simulink model "MRAC_OF_Non_Linear_Simulink"  (R2018a)
settings: Solver=ode45  StartTime=0.0  StopTime=20*T_Uc  RelTol=1e-3  EnableMultiTasking=on
undefined symbols (not defined in the file): a0, a1, a2, A_ch1, A_ch2, A_p, alfa, Am, am1, am2, Amp_Uc, b, b0, b0_init, bm, C, d, Gamma, gamma1, gamma2, h0_1, h0_2, h1_init, h2_init, l, mu, P, P1, P2, P2_init, P_atm, Ps, R, r1p, r1p_init, Roh_air, Roh_w, s0, s0_init, s1, s1_init, T0, t0, t0_init, T1, t1, t1_init, T2, T_Uc, Tf, Ts
settings Model: Creator=ahmad  LastModifiedBy=Ahmad
settings DataIOCC: LimitDataPoints=on  SaveFormat=Array
settings OptimizationCC: LifeSpan=inf
settings DebuggingCC: UnderspecifiedInitializationDetection=Classic  MergeDetectMultiDrivingBlocksExec=none  SolverPrmCheckMsg=warning  StateNameClashWarn=warning  SFUnexpectedBacktrackingDiag=warning  SFNoUnconditionalDefaultTransitionDiag=warning  SFExecutionAtInitializationDiag=none
settings HardwareCC: ProdBitPerPointer=32  ProdBitPerSizeT=32  ProdBitPerPtrDiffT=32  ProdLargestAtomicFloat=None  ProdIntDivRoundTo=Undefined  ProdEndianess=Unspecified  ProdWordSize=32  ProdHWDeviceType=32-bit Generic
settings ModelReferenceCC: PropagateSignalLabelsOutOfModel=off
settings CodeAppCC: StateflowObjectComments=on
settings GRTTargetCC: TargetLangStandard=C89/C90 (ANSI)  GeneratePreprocessorConditionals=Disable all
settings ConfigComp: CovMetricSettings=dw  CovHtmlReporting=on  CovSaveCumulativeToWorkspaceVar=on  CovSaveSingleToWorkspaceVar=on  CovExternalEMLEnable=off

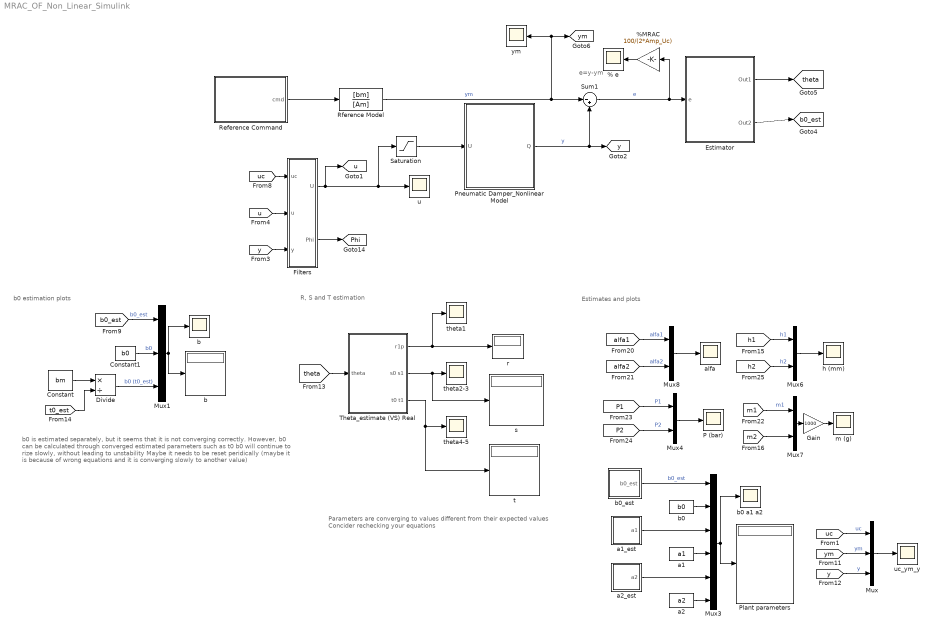
== system MRAC_OF_Non_Linear_Simulink ==
  note: Estimates and plots
  note: R, S and T estimation
  note: b0 estimation plots
  note: Parameters are converging to values different from their expected values
      | Concider rechecking your equations
  note: b0 is estimated separately, but it seems that it is not converging correctly.
      | However, b0 can be calculated through converged estimated parameters such as t0
      |
      | b0 will continue to rize slowly, without leading to unstability
      | Maybe it needs to be reset peridically
      | (maybe it is because of wrong equations and it is converging slowly to another value)
  note: e=y-ym
  % e : Scope
  %MRAC : Gain  Gain=100/(2*Amp_Uc)
  Constant : Constant  Value=bm
  Constant1 : Constant  Value=b0
  Divide : Product  Inputs=*/
  Estimator : Subsystem
  Filters : Subsystem
  Gain : Gain  Gain=1000
  Mux : Mux  Inputs=3
  Mux1 : Mux  Inputs=3
  Mux3 : Mux  Inputs=6
  Mux{4,6..8} (4 alike) : Mux  Inputs=2
  P (bar) : Scope
  Plant parameters : Display
  Pneumatic Damper_Nonlinear Model : Subsystem
  Reference Command : Subsystem
  Rference Model : TransferFcn  Numerator=[bm]  Denominator=[Am]
  Saturation : Saturate  UpperLimit=1  LowerLimit=-1
  Sum1 : Sum  Inputs=|-+
  Theta_estimate (VS) Real : Subsystem
  a1 : Constant  Value=a1
  a1_est : Subsystem
  a2 : Constant  Value=a2
  a2_est : Subsystem
  alfa : Scope
  b : Scope
  "b " : Display
  b0 : Constant  Value=b0
  b0 a1 a2 : Scope
  b0_est : Subsystem
  h (mm) : Scope
  m (g) : Scope
  r : Display
  s : Display
  t : Display
  theta1 : Scope
  theta2-3 : Scope
  theta4-5 : Scope
  u : Scope
  uc_ym_y : Scope
  ym : Scope
  tag scope: Phi=global, b0_est=global, theta=global, u=global, y=global, ym=global
  wires:
  Pneumatic Damper_Nonlinear Model/1("Q  ") -> [y], Sum1/2  "y"
  Rference Model/1 -> Sum1/1, [ym], ym/1  "ym"
  Sum1/1 -> %MRAC/1, Estimator/1(e)  "e"
  Mux/1 -> uc_ym_y/1
  [uc] -> Mux/1  "uc"
  [u] -> Filters/2(u)
  [y] -> Filters/3(y)
  Filters/2(Phi) -> [Phi]
  Mux1/1 -> "b "/1, b/1
  Constant1/1 -> Mux1/2  "b0"
  [b0_est] -> Mux1/1  "b0_est"
  [uc] -> Filters/1(uc)
  Filters/1(U) -> Saturation/1, u/1, [u]
  [y] -> Mux/3  "y"
  [ym] -> Mux/2  "ym"
  Theta_estimate (VS) Real/3(t0	t1) -> t/1, theta4-5/1
  Theta_estimate (VS) Real/2(s0	s1) -> s/1, theta2-3/1
  Theta_estimate (VS) Real/1(r1p) -> theta1/1, r/1
  [theta] -> Theta_estimate (VS) Real/1(theta)
  [t0_est] -> Divide/2
  Constant/1 -> Divide/1
  Divide/1 -> Mux1/3  "b0 (t0_est)"
  Mux3/1 -> b0 a1 a2/1, Plant parameters/1
  b0/1 -> Mux3/2
  a1/1 -> Mux3/4
  b0_est/1(b0_est) -> Mux3/1  "b0_est"
  a1_est/1(a1) -> Mux3/3
  a2_est/1(a2) -> Mux3/5
  a2/1 -> Mux3/6
  %MRAC/1 -> % e/1
  [P1] -> Mux4/1  "P1"
  [P2] -> Mux4/2  "P2"
  Mux4/1 -> P (bar)/1
  [h1] -> Mux6/1  "h1"
  [h2] -> Mux6/2  "h2"
  Mux6/1 -> h (mm)/1
  [m1] -> Mux7/1  "m1"
  [m2] -> Mux7/2
  Mux7/1 -> Gain/1
  Gain/1 -> m (g)/1
  [alfa1] -> Mux8/1  "alfa1"
  [alfa2] -> Mux8/2  "alfa2"
  Mux8/1 -> alfa/1
  Saturation/1 -> Pneumatic Damper_Nonlinear Model/1(U)
  Reference Command/1(cmd) -> Rference Model/1
  Estimator/1(Out1) -> [theta]
  Estimator/2(Out2) -> [b0_est]

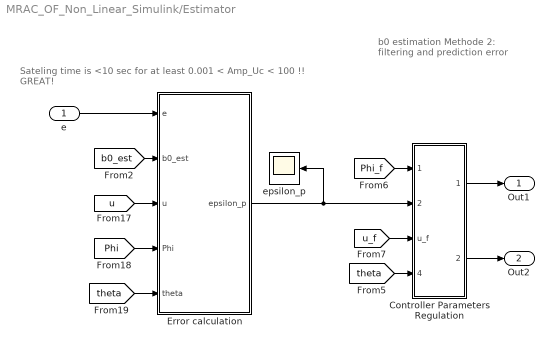
== system MRAC_OF_Non_Linear_Simulink/Estimator ==
  note: b0 estimation
      | Methode 2:
      | filtering and prediction error
  note: Sateling time is <10 sec for at least 0.001 < Amp_Uc < 100 !!
      | GREAT!
  e : Inport
  Controller Parameters Regulation : Subsystem
  Error calculation : Subsystem
  epsilon_p : Scope
  Out1 : Outport
  Out2 : Outport  Port=2
  wires:
  [Phi] -> Error calculation/4("Phi ")
  [b0_est] -> Error calculation/2(b0_est)
  e/1 -> Error calculation/1("e ")
  [u] -> Error calculation/3(u)
  [Phi_f] -> Controller Parameters Regulation/1(Phi_f)
  [u_f] -> Controller Parameters Regulation/3(u_f)
  [theta] -> Error calculation/5(theta)
  Error calculation/1(epsilon_p) -> epsilon_p/1, Controller Parameters Regulation/2(epsilon_p)
  [theta] -> Controller Parameters Regulation/4("theta ")
  Controller Parameters Regulation/2(b0_est) -> Out2/1
  Controller Parameters Regulation/1(theta) -> Out1/1

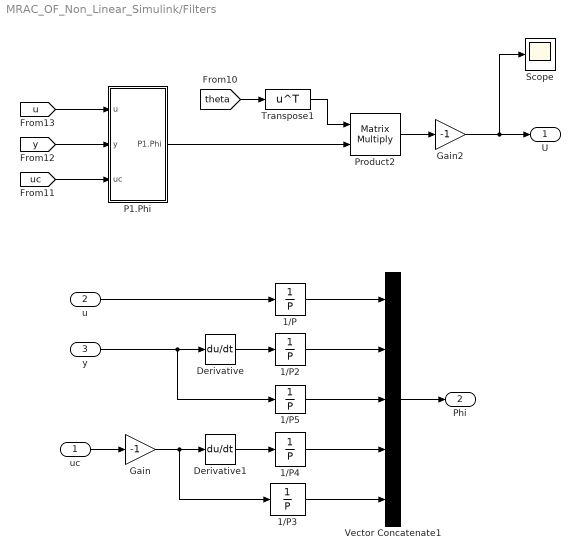
== system MRAC_OF_Non_Linear_Simulink/Filters ==
  uc : Inport
  u : Inport  Port=2
  y : Inport  Port=3
  1/P{,2..5} (5 alike) : TransferFcn  Numerator=1  Denominator=P
  Derivative : Derivative
  Derivative1 : Derivative
  Gain : Gain  Gain=-1
  Gain2 : Gain  Gain=-1
  P1.Phi : Subsystem
  Product2 : Product  Multiplication=Matrix(*)
  Scope : Scope
  Transpose1 : Math  Operator=transpose  SaturateOnIntegerOverflow=on
  Vector Concatenate1 : Concatenate  NumInputs=5
  U : Outport
  Phi : Outport  Port=2
  wires:
  y/1 -> 1/P5/1, Derivative/1
  Derivative1/1 -> 1/P4/1
  1/P3/1 -> Vector Concatenate1/5
  Gain/1 -> 1/P3/1, Derivative1/1
  1/P2/1 -> Vector Concatenate1/2
  Derivative/1 -> 1/P2/1
  1/P4/1 -> Vector Concatenate1/4
  u/1 -> 1/P/1
  Vector Concatenate1/1 -> Phi/1
  1/P5/1 -> Vector Concatenate1/3
  uc/1 -> Gain/1
  1/P/1 -> Vector Concatenate1/1
  [u] -> P1.Phi/1(u)
  [y] -> P1.Phi/2(y)
  [uc] -> P1.Phi/3(uc)
  P1.Phi/1(P1.Phi) -> Product2/2
  Transpose1/1 -> Product2/1
  [theta] -> Transpose1/1
  Product2/1 -> Gain2/1
  Gain2/1 -> Scope/1, U/1

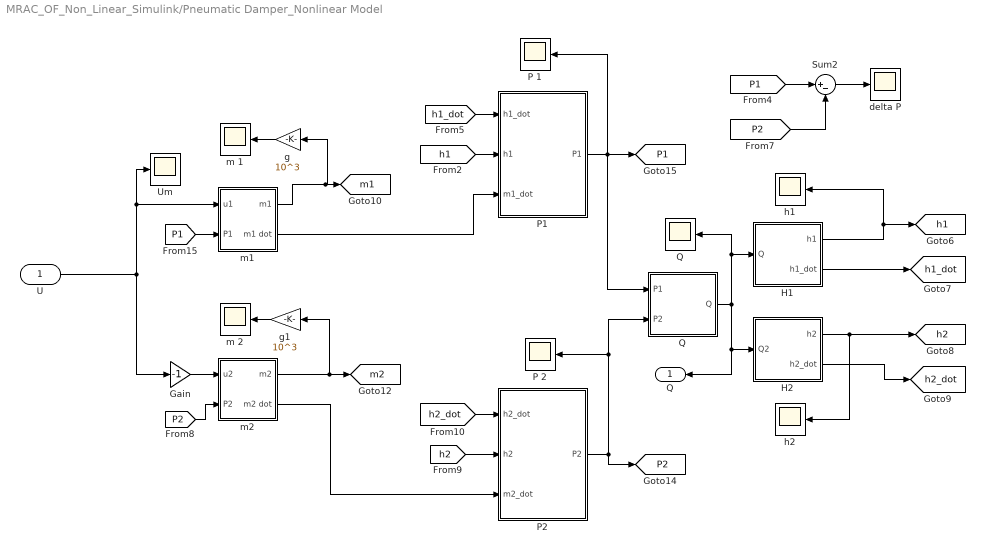
== system MRAC_OF_Non_Linear_Simulink/Pneumatic Damper_Nonlinear Model ==
  U : Inport
  Gain : Gain  Gain=-1
  H1 : Subsystem
  H2 : Subsystem
  P 1 : Scope
  P 2 : Scope
  P1 : Subsystem
  P2 : Subsystem
  Q : Subsystem
  "Q " : Scope
  Sum2 : Sum  Inputs=|+-
  Um : Scope
  delta P : Scope
  g : Gain  Gain=10^3
  g1 : Gain  Gain=10^3
  h1 : Scope
  h2 : Scope
  m 1 : Scope
  m 2 : Scope
  m1 : Subsystem
  m2 : Subsystem
  "Q  " : Outport
  tag scope: P1=global, P2=global, h1=global, h1_dot=global, h2=global, h2_dot=global, m1=global, m2=global
  wires:
  H1/1(h1) -> [h1], h1/1
  H1/2(h1_dot) -> [h1_dot]
  H2/2(h2_dot) -> [h2_dot]
  H2/1(h2) -> h2/1, [h2]
  m1/1(m1) -> g/1, [m1]
  m2/1(m2) -> g1/1, [m2]
  m2/2(m2 dot) -> P2/3(m2_dot)
  [h2_dot] -> P2/1(h2_dot)
  [h1] -> P1/2(h1)
  [h2] -> P2/2(h2)
  P2/1(P2) -> [P2], P 2/1, Q/2(P2)
  U/1 -> Um/1, m1/1(u1), Gain/1
  P1/1(P1) -> P 1/1, Q/1(P1), [P1]
  Gain/1 -> m2/1(u2)
  Q/1(Q) -> "Q  "/1, H2/1(Q2), H1/1(Q), "Q "/1
  [h1_dot] -> P1/1(h1_dot)
  g/1 -> m 1/1
  [P1] -> Sum2/1
  Sum2/1 -> delta P/1
  [P2] -> Sum2/2
  m1/2(m1 dot) -> P1/3(m1_dot)
  [P2] -> m2/2(P2)
  g1/1 -> m 2/1
  [P1] -> m1/2(P1)

== system MRAC_OF_Non_Linear_Simulink/Reference Command ==
  note: without the Uc filter, the parameters do not converge properly!
  note: Assign  Amp_U from the MATLAB script only!
      | gamma and alfa are based on its value!!
  Constant2 : Constant  Value=gamma1
  Constant3 : Constant  Value=alfa
  Input signal (Uc) : DiscretePulseGenerator  PulseType=Time based  Amplitude=-Amp_Uc  Period=T_Uc  PulseWidth=50  PhaseDelay=T_Uc/2
  "Input signal (Uc) Amp_Uc T_uc " : DiscretePulseGenerator  PulseType=Time based  Amplitude=Amp_Uc  Period=T_Uc  PulseWidth=50
  Mux2 : Mux  Inputs=2
  Sum2 : Sum  Inputs=|++
  Uc filter : TransferFcn  Denominator=conv(conv([T_Uc/100 1],[T_Uc/100 1]),[T_Uc/100 1])
  gamma alfa : Display
  uc : Scope
  cmd : Outport
  tag scope: uc=global
  wires:
  Constant2/1 -> Mux2/1
  Input signal (Uc)/1 -> Sum2/1
  Mux2/1 -> gamma alfa/1
  Uc filter/1 -> cmd/1, [uc], uc/1
  Constant3/1 -> Mux2/2
  Sum2/1 -> Uc filter/1
  "Input signal (Uc) Amp_Uc T_uc "/1 -> Sum2/2

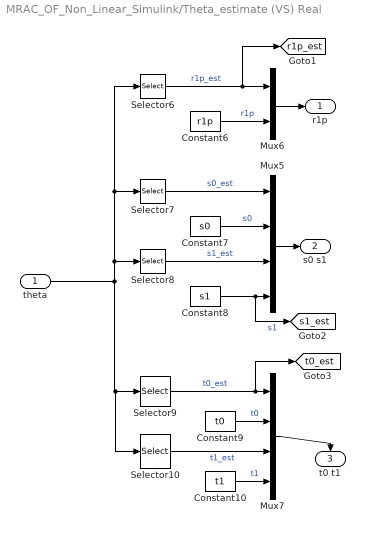
== system MRAC_OF_Non_Linear_Simulink/Theta_estimate (VS) Real ==
  theta : Inport
  Constant10 : Constant  Value=t1
  Constant6 : Constant  Value=r1p
  Constant7 : Constant  Value=s0
  Constant8 : Constant  Value=s1
  Constant9 : Constant  Value=t0
  Mux5 : Mux
  Mux6 : Mux  Inputs=2
  Mux7 : Mux
  Selector10 : Selector  InputPortWidth=5  IndexOptions=Index vector (dialog)  Indices=[5]  OutputSizes=1
  Selector6 : Selector  InputPortWidth=5  IndexOptions=Index vector (dialog)  Indices=[1]  OutputSizes=1
  Selector7 : Selector  InputPortWidth=5  IndexOptions=Index vector (dialog)  Indices=[2]  OutputSizes=1
  Selector8 : Selector  InputPortWidth=5  IndexOptions=Index vector (dialog)  Indices=[3]  OutputSizes=1
  Selector9 : Selector  InputPortWidth=5  IndexOptions=Index vector (dialog)  Indices=[4]  OutputSizes=1
  r1p : Outport
  s0	s1 : Outport  Port=2
  t0	t1 : Outport  Port=3
  tag scope: r1p_est=global, s1_est=global, t0_est=global
  wires:
  Selector7/1 -> Mux5/1  "s0_est"
  Selector6/1 -> [r1p_est], Mux6/1  "r1p_est"
  Mux5/1 -> s0	s1/1
  Selector8/1 -> Mux5/3  "s1_est"
  Constant8/1 -> [s1_est], Mux5/4  "s1"
  Selector9/1 -> [t0_est], Mux7/1  "t0_est"
  Selector10/1 -> Mux7/3  "t1_est"
  Constant10/1 -> Mux7/4  "t1"
  Mux7/1 -> t0	t1/1
  Constant6/1 -> Mux6/2  "r1p"
  theta/1 -> Selector8/1, Selector6/1, Selector7/1, Selector10/1, Selector9/1
  Constant7/1 -> Mux5/2  "s0"
  Constant9/1 -> Mux7/2  "t0"
  Mux6/1 -> r1p/1

== system MRAC_OF_Non_Linear_Simulink/a1_est ==
  Constant4 : Constant  Value=am1
  Sum2 : Sum  Inputs=|-+
  a1 : Outport
  wires:
  Constant4/1 -> Sum2/2
  [r1p_est] -> Sum2/1
  Sum2/1 -> a1/1  "a1"

== system MRAC_OF_Non_Linear_Simulink/a2_est ==
  Constant1 : Constant  Value=am2*a0
  Constant4 : Constant  Value=a0
  Divide1 : Product  Inputs=**
  Divide2 : Product  Inputs=*/
  Sum1 : Sum  Inputs=|+-
  Sum2 : Sum  Inputs=|++
  a2 : Outport
  wires:
  Constant4/1 -> Sum2/2
  [r1p_est] -> Sum2/1
  [s1_est] -> Divide1/1
  [b0_t0_est] -> Divide1/2
  Divide1/1 -> Sum1/2
  Constant1/1 -> Sum1/1
  Sum1/1 -> Divide2/1
  Sum2/1 -> Divide2/2  "r1"
  Divide2/1 -> a2/1  "a2"

== system MRAC_OF_Non_Linear_Simulink/b0_est ==
  Constant4 : Constant  Value=bm
  Divide1 : Product  Inputs=*/
  b0_est : Outport
  tag scope: b0_t0_est=global
  wires:
  [t0_est] -> Divide1/2
  Divide1/1 -> [b0_t0_est], b0_est/1  "b0 (t0_est)"
  Constant4/1 -> Divide1/1

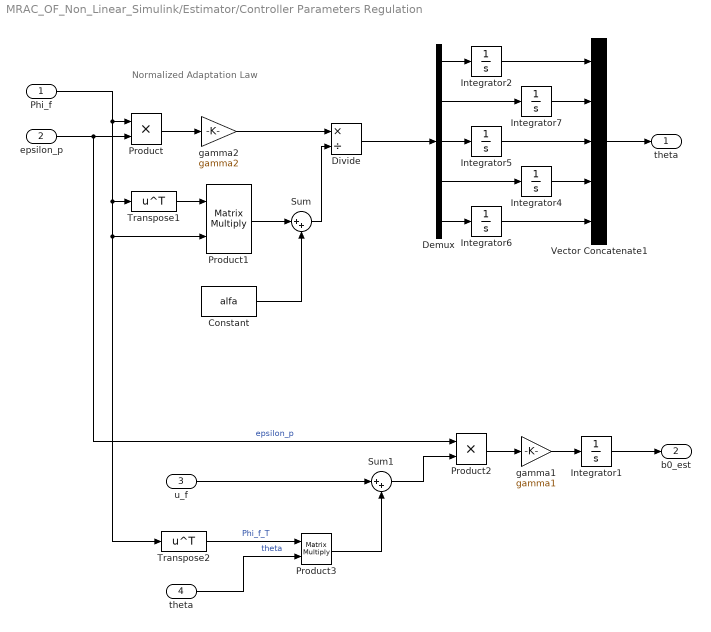
== system MRAC_OF_Non_Linear_Simulink/Estimator/Controller Parameters Regulation ==
  note: Normalized Adaptation Law
  Phi_f : Inport
  epsilon_p : Inport  Port=2
  u_f : Inport  Port=3
  "theta " : Inport  Port=4
  Constant : Constant  Value=alfa
  Demux : Demux  Outputs=5
  Divide : Product  Inputs=*/
  Integrator1 : Integrator  InitialCondition=b0_init
  Integrator2 : Integrator  InitialCondition=r1p_init
  Integrator4 : Integrator  InitialCondition=t0_init
  Integrator5 : Integrator  InitialCondition=s1_init
  Integrator6 : Integrator  InitialCondition=t1_init
  Integrator7 : Integrator  InitialCondition=s0_init
  Product : Product
  Product1 : Product  Multiplication=Matrix(*)
  Product2 : Product
  Product3 : Product  Multiplication=Matrix(*)
  Sum : Sum  Inputs=|++
  Sum1 : Sum  Inputs=|++
  Transpose1 : Math  Operator=transpose  SaturateOnIntegerOverflow=on
  Transpose2 : Math  Operator=transpose  SaturateOnIntegerOverflow=on
  Vector Concatenate1 : Concatenate  NumInputs=5
  gamma1 : Gain  Gain=gamma1
  "gamma2 " : Gain  Gain=gamma2
  theta : Outport
  b0_est : Outport  Port=2
  wires:
  Integrator2/1 -> Vector Concatenate1/1
  Vector Concatenate1/1 -> theta/1
  epsilon_p/1 -> Product2/1, Product/2  "epsilon_p"
  "gamma2 "/1 -> Divide/1
  Demux/4 -> Integrator4/1
  Demux/5 -> Integrator6/1
  Integrator5/1 -> Vector Concatenate1/3
  Integrator4/1 -> Vector Concatenate1/4
  Demux/3 -> Integrator5/1
  Integrator7/1 -> Vector Concatenate1/2
  Integrator6/1 -> Vector Concatenate1/5
  Demux/1 -> Integrator2/1
  Demux/2 -> Integrator7/1
  Phi_f/1 -> Transpose2/1, Product1/2, Transpose1/1, Product/1
  Product/1 -> "gamma2 "/1
  Transpose1/1 -> Product1/1
  Product1/1 -> Sum/1
  Constant/1 -> Sum/2
  Sum/1 -> Divide/2
  Divide/1 -> Demux/1
  u_f/1 -> Sum1/1
  Product2/1 -> gamma1/1
  gamma1/1 -> Integrator1/1
  Integrator1/1 -> b0_est/1
  Transpose2/1 -> Product3/1  "Phi_f_T"
  "theta "/1 -> Product3/2  "theta"
  Product3/1 -> Sum1/2
  Sum1/1 -> Product2/2

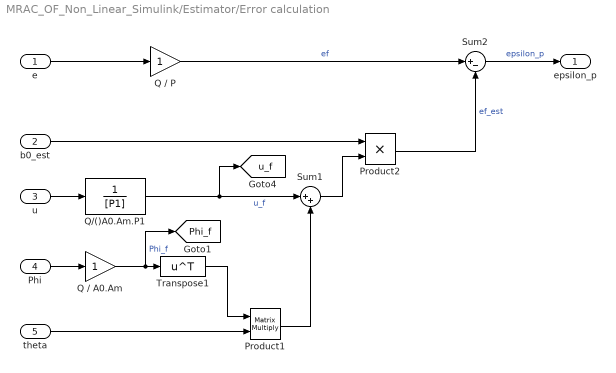
== system MRAC_OF_Non_Linear_Simulink/Estimator/Error calculation ==
  "e " : Inport
  b0_est : Inport  Port=2
  u : Inport  Port=3
  "Phi " : Inport  Port=4
  theta : Inport  Port=5
  Product1 : Product  Multiplication=Matrix(*)
  Product2 : Product
  "Q / A0.Am " : Gain
  Q / P : Gain
  Q/()A0.Am.P1 : TransferFcn  Denominator=[P1]
  Sum1 : Sum  Inputs=|++
  Sum2 : Sum  Inputs=|+-
  Transpose1 : Math  Operator=transpose  SaturateOnIntegerOverflow=on
  epsilon_p : Outport
  tag scope: Phi_f=global, u_f=global
  wires:
  "e "/1 -> Q / P/1
  Q / P/1 -> Sum2/1  "ef"
  Sum2/1 -> epsilon_p/1  "epsilon_p"
  b0_est/1 -> Product2/1
  u/1 -> Q/()A0.Am.P1/1
  Q/()A0.Am.P1/1 -> [u_f], Sum1/1  "u_f"
  "Phi "/1 -> "Q / A0.Am "/1
  "Q / A0.Am "/1 -> [Phi_f], Transpose1/1  "Phi_f"
  Transpose1/1 -> Product1/1
  theta/1 -> Product1/2
  Product1/1 -> Sum1/2
  Sum1/1 -> Product2/2
  Product2/1 -> Sum2/2  "ef_est"

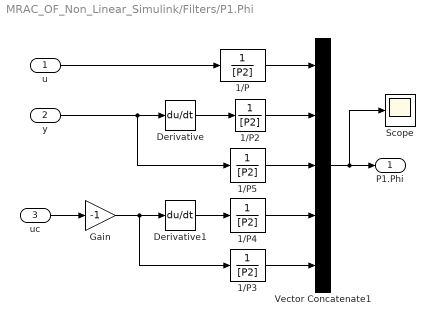
== system MRAC_OF_Non_Linear_Simulink/Filters/P1.Phi ==
  u : Inport
  y : Inport  Port=2
  uc : Inport  Port=3
  1/P{,2..5} (5 alike) : TransferFcn  Numerator=1  Denominator=[P2]
  Derivative : Derivative
  Derivative1 : Derivative
  Gain : Gain  Gain=-1
  Scope : Scope
  Vector Concatenate1 : Concatenate  NumInputs=5
  P1.Phi : Outport
  wires:
  y/1 -> 1/P5/1, Derivative/1
  Derivative1/1 -> 1/P4/1
  1/P3/1 -> Vector Concatenate1/5
  Gain/1 -> 1/P3/1, Derivative1/1
  1/P2/1 -> Vector Concatenate1/2
  Derivative/1 -> 1/P2/1
  1/P4/1 -> Vector Concatenate1/4
  u/1 -> 1/P/1
  1/P5/1 -> Vector Concatenate1/3
  uc/1 -> Gain/1
  1/P/1 -> Vector Concatenate1/1
  Vector Concatenate1/1 -> Scope/1, P1.Phi/1

== system MRAC_OF_Non_Linear_Simulink/Pneumatic Damper_Nonlinear Model/H1 ==
  Q : Inport
  Constant : Constant  Value=A_ch1
  Divide : Product  Inputs=*/
  Integrator : Integrator  InitialCondition=h1_init
  cm-mm : Gain  Gain=-10^3
  h1 : Outport
  h1_dot : Outport  Port=2
  wires:
  Q/1 -> Divide/1
  Integrator/1 -> h1/1  "h1"
  cm-mm/1 -> h1_dot/1, Integrator/1  "h1_dot"
  Divide/1 -> cm-mm/1
  Constant/1 -> Divide/2

== system MRAC_OF_Non_Linear_Simulink/Pneumatic Damper_Nonlinear Model/H2 ==
  Q2 : Inport
  A_pressure_chamber2 : Constant  Value=A_ch2
  Divide : Product  Inputs=*/
  Integrator : Integrator  InitialCondition=h2_init
  cm-mm : Gain  Gain=10^3
  h2 : Outport
  h2_dot : Outport  Port=2
  wires:
  A_pressure_chamber2/1 -> Divide/2
  Q2/1 -> Divide/1
  Integrator/1 -> h2/1  "h2"
  Divide/1 -> cm-mm/1  "h2_dot"
  cm-mm/1 -> Integrator/1, h2_dot/1

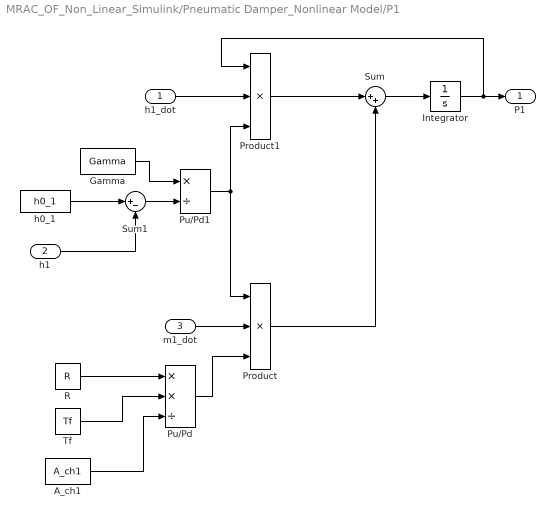
== system MRAC_OF_Non_Linear_Simulink/Pneumatic Damper_Nonlinear Model/P1 ==
  h1_dot : Inport
  h1 : Inport  Port=2
  m1_dot : Inport  Port=3
  A_ch1 : Constant  Value=A_ch1
  Gamma : Constant  Value=Gamma
  Integrator : Integrator  InitialCondition=P2_init
  Product : Product  Inputs=3
  Product1 : Product  Inputs=3
  Pu/Pd : Product  Inputs=**/
  Pu/Pd1 : Product  Inputs=*/
  R : Constant  Value=R
  Sum : Sum  Inputs=|++
  Sum1 : Sum  Inputs=|+-
  Tf : Constant  Value=Tf
  h0_1 : Constant  Value=h0_1
  P1 : Outport
  wires:
  R/1 -> Pu/Pd/1
  A_ch1/1 -> Pu/Pd/3
  Gamma/1 -> Pu/Pd1/1
  Sum1/1 -> Pu/Pd1/2
  h0_1/1 -> Sum1/1
  Tf/1 -> Pu/Pd/2
  Pu/Pd1/1 -> Product/1, Product1/3
  Pu/Pd/1 -> Product/3
  Sum/1 -> Integrator/1
  Integrator/1 -> Product1/1, P1/1
  Product1/1 -> Sum/1
  Product/1 -> Sum/2
  h1_dot/1 -> Product1/2
  h1/1 -> Sum1/2
  m1_dot/1 -> Product/2

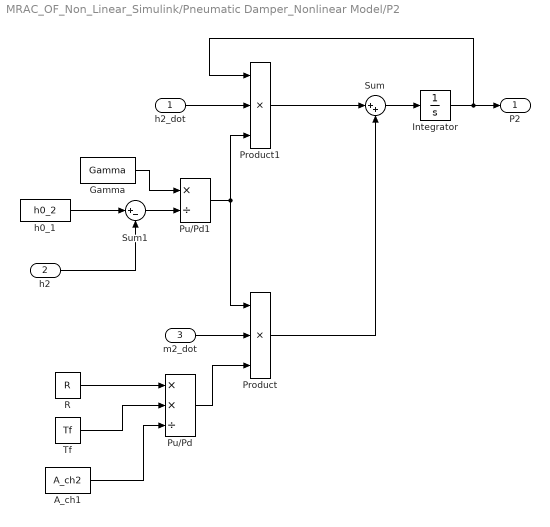
== system MRAC_OF_Non_Linear_Simulink/Pneumatic Damper_Nonlinear Model/P2 ==
  h2_dot : Inport
  h2 : Inport  Port=2
  m2_dot : Inport  Port=3
  A_ch1 : Constant  Value=A_ch2
  Gamma : Constant  Value=Gamma
  Integrator : Integrator  InitialCondition=P2_init
  Product : Product  Inputs=3
  Product1 : Product  Inputs=3
  Pu/Pd : Product  Inputs=**/
  Pu/Pd1 : Product  Inputs=*/
  R : Constant  Value=R
  Sum : Sum  Inputs=|++
  Sum1 : Sum  Inputs=|+-
  Tf : Constant  Value=Tf
  h0_1 : Constant  Value=h0_2
  P2 : Outport
  wires:
  R/1 -> Pu/Pd/1
  A_ch1/1 -> Pu/Pd/3
  Integrator/1 -> Product1/1, P2/1
  Gamma/1 -> Pu/Pd1/1
  Sum1/1 -> Pu/Pd1/2
  h0_1/1 -> Sum1/1
  Tf/1 -> Pu/Pd/2
  Pu/Pd1/1 -> Product/1, Product1/3
  Pu/Pd/1 -> Product/3
  Sum/1 -> Integrator/1
  Product1/1 -> Sum/1
  Product/1 -> Sum/2
  h2_dot/1 -> Product1/2
  h2/1 -> Sum1/2
  m2_dot/1 -> Product/2

== system MRAC_OF_Non_Linear_Simulink/Pneumatic Damper_Nonlinear Model/Q ==
  P1 : Inport
  P2 : Inport  Port=2
  Integrator : Integrator
  Product1 : Product
  Product2 : Product
  Q 2 : Scope
  Sum : Sum  Inputs=|+-
  Sum1 : Sum  Inputs=|+-
  c 4 : Gain  Gain=10^8
  c 5 : Gain  Gain=10^11
  c4 : Subsystem
  c5 : Subsystem
  Q : Outport
  wires:
  P1/1 -> Sum/1
  P2/1 -> Sum/2
  Sum/1 -> Product1/2
  Product1/1 -> Sum1/1
  Integrator/1 -> Q 2/1, Product2/2, Q/1  "Q"
  Product2/1 -> Sum1/2
  Sum1/1 -> Integrator/1
  c4/1(c4) -> c 4/1
  c 4/1 -> Product1/1
  c 5/1 -> Product2/1
  c5/1(c5) -> c 5/1

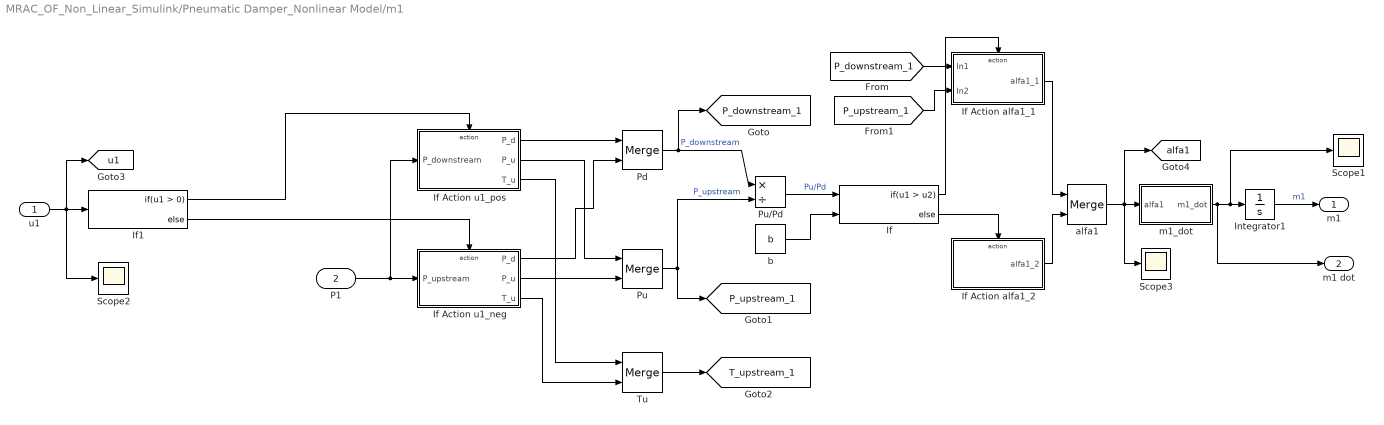
== system MRAC_OF_Non_Linear_Simulink/Pneumatic Damper_Nonlinear Model/m1 ==
  u1 : Inport
  P1 : Inport  Port=2
  If : If  NumInputs=2  IfExpression=u1 > u2
  If Action alfa1_1 : Subsystem  TreatAsAtomicUnit=on
  If Action alfa1_2 : Subsystem  TreatAsAtomicUnit=on
  If Action u1_neg : Subsystem  TreatAsAtomicUnit=on
  If Action u1_pos : Subsystem  TreatAsAtomicUnit=on
  If1 : If
  Integrator1 : Integrator
  Pd : Merge
  Pu : Merge
  Pu/Pd : Product  Inputs=*/
  Scope1 : Scope
  Scope2 : Scope
  Scope3 : Scope
  Tu : Merge
  alfa1 : Merge
  b : Constant  Value=b
  m1_dot : Subsystem
  m1 : Outport
  m1 dot : Outport  Port=2
  tag scope: P_downstream_1=global, P_upstream_1=global, T_upstream_1=global, alfa1=global, u1=global
  wires:
  alfa1/1 -> [alfa1], Scope3/1, m1_dot/1(alfa1)
  Integrator1/1 -> m1/1  "m1"
  If1/2 -> If Action u1_neg/Action
  u1/1 -> Scope2/1, [u1], If1/1
  If1/1 -> If Action u1_pos/Action
  Pu/Pd/1 -> If/1  "Pu/Pd"
  If/1 -> If Action alfa1_1/Action
  If/2 -> If Action alfa1_2/Action
  b/1 -> If/2
  Pd/1 -> Pu/Pd/1, [P_downstream_1]  "P_downstream"
  Pu/1 -> Pu/Pd/2, [P_upstream_1]  "P_upstream"
  If Action u1_pos/1(P_d) -> Pd/1
  If Action alfa1_2/1(alfa1_2) -> alfa1/2
  If Action alfa1_1/1(alfa1_1) -> alfa1/1
  If Action u1_neg/1(P_d) -> Pd/2
  If Action u1_pos/2(P_u) -> Pu/1
  If Action u1_neg/2(P_u) -> Pu/2
  m1_dot/1(m1_dot) -> m1 dot/1, Scope1/1, Integrator1/1
  If Action u1_neg/3(T_u) -> Tu/2
  If Action u1_pos/3(T_u) -> Tu/1
  Tu/1 -> [T_upstream_1]
  [P_downstream_1] -> If Action alfa1_1/1(In1)
  [P_upstream_1] -> If Action alfa1_1/2(In2)
  P1/1 -> If Action u1_pos/1(P_downstream), If Action u1_neg/1(P_upstream)

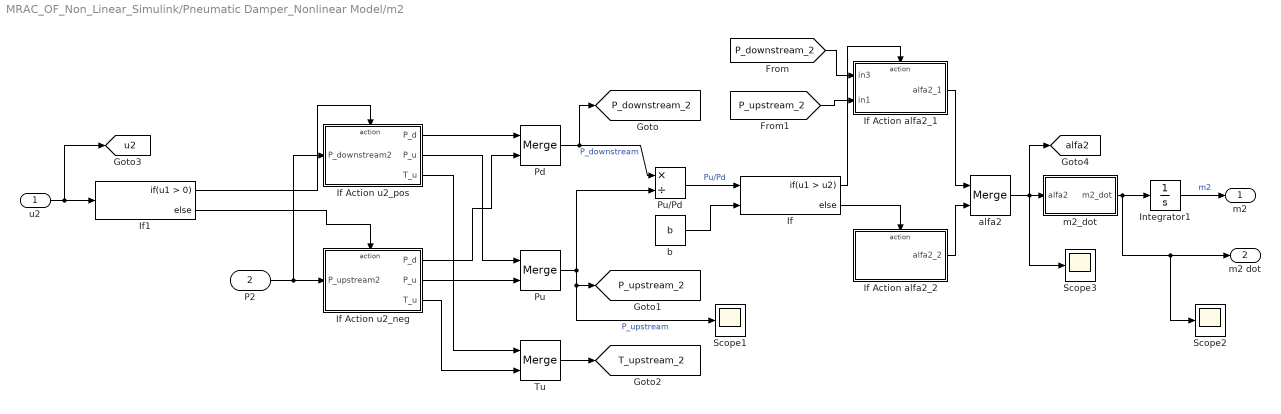
== system MRAC_OF_Non_Linear_Simulink/Pneumatic Damper_Nonlinear Model/m2 ==
  u2 : Inport
  P2 : Inport  Port=2
  If : If  NumInputs=2  IfExpression=u1 > u2
  If Action alfa2_1 : Subsystem  TreatAsAtomicUnit=on
  If Action alfa2_2 : Subsystem  TreatAsAtomicUnit=on
  If Action u2_neg : Subsystem  TreatAsAtomicUnit=on
  If Action u2_pos : Subsystem  TreatAsAtomicUnit=on
  If1 : If
  Integrator1 : Integrator
  Pd : Merge
  Pu : Merge
  Pu/Pd : Product  Inputs=*/
  Scope1 : Scope
  Scope2 : Scope
  Scope3 : Scope
  Tu : Merge
  alfa2 : Merge
  b : Constant  Value=b
  m2_dot : Subsystem
  m2 : Outport
  m2 dot : Outport  Port=2
  tag scope: P_downstream_2=global, P_upstream_2=global, T_upstream_2=global, alfa2=global, u2=global
  wires:
  alfa2/1 -> [alfa2], Scope3/1, m2_dot/1(alfa2)
  Integrator1/1 -> m2/1  "m2"
  If1/2 -> If Action u2_neg/Action
  u2/1 -> [u2], If1/1
  If1/1 -> If Action u2_pos/Action
  Pu/Pd/1 -> If/1  "Pu/Pd"
  If/1 -> If Action alfa2_1/Action
  If/2 -> If Action alfa2_2/Action
  b/1 -> If/2
  Pd/1 -> [P_downstream_2], Pu/Pd/1  "P_downstream"
  Pu/1 -> Pu/Pd/2, Scope1/1, [P_upstream_2]  "P_upstream"
  If Action u2_pos/1(P_d) -> Pd/1
  If Action alfa2_2/1(alfa2_2) -> alfa2/2
  If Action alfa2_1/1(alfa2_1) -> alfa2/1
  If Action u2_neg/1(P_d) -> Pd/2
  If Action u2_pos/2(P_u) -> Pu/1
  If Action u2_neg/2(P_u) -> Pu/2
  m2_dot/1(m2_dot) -> Scope2/1, m2 dot/1, Integrator1/1
  If Action u2_neg/3(T_u) -> Tu/2
  If Action u2_pos/3(T_u) -> Tu/1
  Tu/1 -> [T_upstream_2]
  P2/1 -> If Action u2_neg/1(P_upstream2), If Action u2_pos/1(P_downstream2)
  [P_downstream_2] -> If Action alfa2_1/1(in3)
  [P_upstream_2] -> If Action alfa2_1/2(in1)

== system MRAC_OF_Non_Linear_Simulink/Pneumatic Damper_Nonlinear Model/Q/c4 ==
  Constant1 : Constant  Value=A_p
  Constant2 : Constant  Value=Roh_w
  Constant3 : Constant  Value=l
  Divide1 : Product  Inputs=*//
  Sum : Sum  Inputs=|++
  c4 : Outport
  wires:
  Constant1/1 -> Divide1/1
  Constant2/1 -> Divide1/3
  Constant3/1 -> Sum/1
  Divide1/1 -> c4/1
  Sum/1 -> Divide1/2
  [l_change] -> Sum/2

== system MRAC_OF_Non_Linear_Simulink/Pneumatic Damper_Nonlinear Model/Q/c5 ==
  Constant4 : Constant  Value=mu
  Constant5 : Constant  Value=A_p
  Constant6 : Constant  Value=Roh_w
  Constant7 : Constant  Value=d^4
  Gain1 : Gain  Gain=128/pi
  Pu/Pd : Product  Inputs=**//
  c5 : Outport
  wires:
  Gain1/1 -> c5/1
  Pu/Pd/1 -> Gain1/1
  Constant4/1 -> Pu/Pd/1
  Constant6/1 -> Pu/Pd/3
  Constant5/1 -> Pu/Pd/2
  Constant7/1 -> Pu/Pd/4

== system MRAC_OF_Non_Linear_Simulink/Pneumatic Damper_Nonlinear Model/m1/If Action alfa1_1 ==
  note: Pu
  In1 : Inport
  In2 : Inport  Port=2
  Action Port : ActionPort  ActionType=then
  Mux : Mux  Inputs=3
  alfa : Fcn  Expr=sqrt(1-((u(1)/u(2)-u(3))/(1-u(3)))^2)
  b : Constant  Value=b
  alfa1_1 : Outport
  wires:
  b/1 -> Mux/3
  Mux/1 -> alfa/1
  In1/1 -> Mux/1  "Pd"
  In2/1 -> Mux/2
  alfa/1 -> alfa1_1/1

== system MRAC_OF_Non_Linear_Simulink/Pneumatic Damper_Nonlinear Model/m1/If Action alfa1_2 ==
  Action Port : ActionPort  ActionType=else
  alfa : Constant
  alfa1_2 : Outport
  wires:
  alfa/1 -> alfa1_2/1

== system MRAC_OF_Non_Linear_Simulink/Pneumatic Damper_Nonlinear Model/m1/If Action u1_neg ==
  P_upstream : Inport
  Action Port : ActionPort  ActionType=else
  P_downstream : Constant  Value=P_atm
  T_upstream : Constant  Value=T1
  P_d : Outport
  P_u : Outport  Port=2
  T_u : Outport  Port=3
  wires:
  P_upstream/1 -> P_u/1
  P_downstream/1 -> P_d/1
  T_upstream/1 -> T_u/1

== system MRAC_OF_Non_Linear_Simulink/Pneumatic Damper_Nonlinear Model/m1/If Action u1_pos ==
  P_downstream : Inport
  Action Port : ActionPort  ActionType=then
  P_upstream : Constant  Value=Ps
  T_upstream : Constant  Value=Ts
  P_d : Outport
  P_u : Outport  Port=2
  T_u : Outport  Port=3
  wires:
  P_upstream/1 -> P_u/1
  P_downstream/1 -> P_d/1
  T_upstream/1 -> T_u/1

== system MRAC_OF_Non_Linear_Simulink/Pneumatic Damper_Nonlinear Model/m1/m1_dot ==
  alfa1 : Inport
  Constant : Constant  Value=C
  Constant2 : Constant  Value=Roh_air
  Constant3 : Constant  Value=T0
  Fcn : Fcn  Expr=sqrt(u(1)/u(2))
  Mux : Mux  Inputs=2
  Product : Product  Inputs=6
  Scope1 : Scope
  Scope2 : Scope
  m1_dot : Outport
  wires:
  Product/1 -> Scope1/1, m1_dot/1
  [P_upstream_1] -> Product/3
  Constant3/1 -> Mux/1
  alfa1/1 -> Product/6
  Fcn/1 -> Product/5
  Mux/1 -> Fcn/1
  Constant2/1 -> Product/4
  [T_upstream_1] -> Mux/2
  [u1] -> Scope2/1, Product/1
  Constant/1 -> Product/2

== system MRAC_OF_Non_Linear_Simulink/Pneumatic Damper_Nonlinear Model/m2/If Action alfa2_1 ==
  note: Pu
  in3 : Inport
  in1 : Inport  Port=2
  Action Port : ActionPort  ActionType=then
  Mux : Mux  Inputs=3
  alfa : Fcn  Expr=sqrt(1-((u(1)/u(2)-u(3))/(1-u(3)))^2)
  b : Constant  Value=b
  alfa2_1 : Outport
  wires:
  b/1 -> Mux/3
  Mux/1 -> alfa/1
  in3/1 -> Mux/1  "Pd"
  in1/1 -> Mux/2
  alfa/1 -> alfa2_1/1

== system MRAC_OF_Non_Linear_Simulink/Pneumatic Damper_Nonlinear Model/m2/If Action alfa2_2 ==
  Action Port : ActionPort  ActionType=else
  alfa : Constant
  alfa2_2 : Outport
  wires:
  alfa/1 -> alfa2_2/1

== system MRAC_OF_Non_Linear_Simulink/Pneumatic Damper_Nonlinear Model/m2/If Action u2_neg ==
  P_upstream2 : Inport
  Action Port : ActionPort  ActionType=else
  P_downstream2 : Constant  Value=P_atm
  T_upstream2 : Constant  Value=T2
  P_d : Outport
  P_u : Outport  Port=2
  T_u : Outport  Port=3
  wires:
  P_upstream2/1 -> P_u/1
  P_downstream2/1 -> P_d/1
  T_upstream2/1 -> T_u/1

== system MRAC_OF_Non_Linear_Simulink/Pneumatic Damper_Nonlinear Model/m2/If Action u2_pos ==
  P_downstream2 : Inport
  Action Port : ActionPort  ActionType=then
  P_upstream2 : Constant  Value=Ps
  T_upstream : Constant  Value=Ts
  P_d : Outport
  P_u : Outport  Port=2
  T_u : Outport  Port=3
  wires:
  P_upstream2/1 -> P_u/1
  P_downstream2/1 -> P_d/1
  T_upstream/1 -> T_u/1

== system MRAC_OF_Non_Linear_Simulink/Pneumatic Damper_Nonlinear Model/m2/m2_dot ==
  alfa2 : Inport
  Constant : Constant  Value=C
  Constant2 : Constant  Value=Roh_air
  Constant3 : Constant  Value=T0
  Fcn : Fcn  Expr=sqrt(u(1)/u(2))
  Mux : Mux  Inputs=2
  Product : Product  Inputs=6
  m2_dot : Outport
  wires:
  Product/1 -> m2_dot/1
  [P_upstream_2] -> Product/3
  Constant3/1 -> Mux/1
  alfa2/1 -> Product/6
  Fcn/1 -> Product/5
  Mux/1 -> Fcn/1
  Constant2/1 -> Product/4
  [T_upstream_2] -> Mux/2
  [u2] -> Product/1
  Constant/1 -> Product/2
